simulink subsystem "Output_Selector_Simple"  (R2021a)
settings: Solver=VariableStepAuto  StartTime=0.0  StopTime=10.0  RelTol=1e-3
libraries: hdlBasic x3
settings Model: Creator=ckk5  LastModifiedBy=ckk5

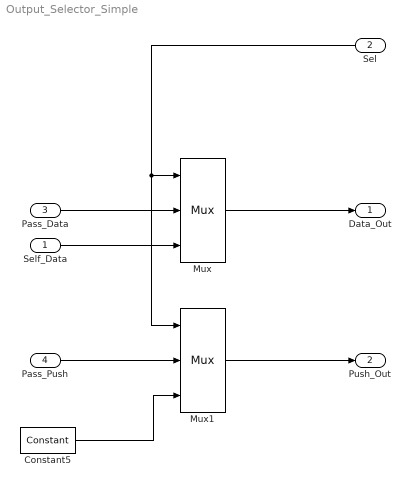
== system Output_Selector_Simple ==
  Self_Data : Inport
  Sel : Inport  Port=2
  Pass_Data : Inport  Port=3
  Pass_Push : Inport  Port=4
  Constant5 : hdlBasic/Constant  const=1  gui_display_data_type=Boolean  arith_type=Boolean  n_bits=16  bin_pt=12  preci_type=Single  exp_width=8  frac_width=24  explicit_period=off  period=1  XmcBlockStatus=1  maskContainerNames=tabcontainer1  block_type=constant  block_config=sysgen:Constant_config
  Mux : hdlBasic/Mux  inputs=2  en=off  latency=1  precision=Full  arith_type=Unsigned  n_bits=16  bin_pt=14  quantization=Truncate  overflow=Wrap  XmcBlockStatus=1  maskContainerNames=tabcontainer1  block_type=mux  block_config=sysgen:Mux_config
  Mux1 : hdlBasic/Mux  inputs=2  en=off  latency=1  precision=Full  arith_type=Unsigned  n_bits=16  bin_pt=14  quantization=Truncate  overflow=Wrap  XmcBlockStatus=1  maskContainerNames=tabcontainer1  block_type=mux  block_config=sysgen:Mux_config
  Data_Out : Outport
  Push_Out : Outport  Port=2
  wires:
  Self_Data/1 -> Mux/3
  Mux/1 -> Data_Out/1
  Pass_Push/1 -> Mux1/2
  Sel/1 -> Mux/1, Mux1/1
  Constant5/1 -> Mux1/3
  Pass_Data/1 -> Mux/2
  Mux1/1 -> Push_Out/1
